simulink model "reaction_wheel"  (R2015b)
settings: Solver=VariableStepAuto  StartTime=0.0  StopTime=500  FixedStep=0.0005  RelTol=1e-3
settings Model: Creator=150010037  LastModifiedBy=150010037

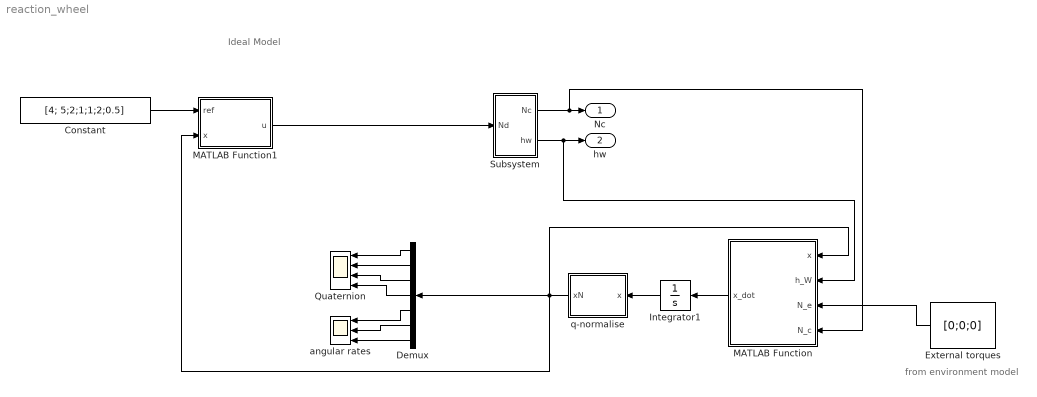
== system reaction_wheel ==
  note: Ideal Model
  note: from environment model
  Constant : Constant  Value=[4; 5;2;1;1;2;0.5]
  Demux : Demux  Outputs=7
  "External torques " : Constant  Value=[0;0;0]
  Integrator1 : Integrator  InitialCondition=[2;3;5;3;0.23;0.5;0.001]
  MATLAB Function : MATLAB Function  TreatAsAtomicUnit=on
  MATLAB Function1 : MATLAB Function  TreatAsAtomicUnit=on
  Quaternion : Scope  NumInputPorts=4
  Subsystem : Subsystem
  angular rates : Scope  NumInputPorts=3
  q-normalise : MATLAB Function  TreatAsAtomicUnit=on
  Nc : Outport
  "hw " : Outport  Port=2
  wires:
  MATLAB Function/1(x_dot) -> Integrator1/1
  Integrator1/1 -> q-normalise/1(x)
  q-normalise/1(xN) -> MATLAB Function1/2(x), MATLAB Function/1(x), Demux/1
  Subsystem/1(Nc) -> MATLAB Function/4(N_c), Nc/1
  Subsystem/2("hw ") -> MATLAB Function/2(h_W), "hw "/1
  "External torques "/1 -> MATLAB Function/3(N_e)
  MATLAB Function1/1(u) -> Subsystem/1(Nd)
  Demux/4 -> Quaternion/4
  Demux/1 -> Quaternion/1
  Demux/2 -> Quaternion/2
  Demux/3 -> Quaternion/3
  Demux/6 -> angular rates/2
  Demux/5 -> angular rates/1
  Demux/7 -> angular rates/3
  Constant/1 -> MATLAB Function1/1(ref)

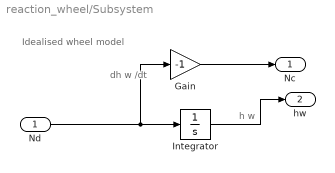
== system reaction_wheel/Subsystem ==
  note: Idealised wheel
      | model
  note: dh w /dt
  note: h w
  Nd : Inport
  Gain : Gain  Gain=-1
  Integrator : Integrator  InitialCondition=[0;0;0]
  Nc : Outport
  "hw " : Outport  Port=2
  wires:
  Nd/1 -> Gain/1, Integrator/1
  Integrator/1 -> "hw "/1
  Gain/1 -> Nc/1

== matlab function reaction_wheel/MATLAB Function1 ==
  data: ref input; x input; u output
function u = fcn(ref,x)
r=ref;
%quaternion error calculation
q_ref=[r(4) r(3) -r(2) -r(1) ;-r(3) r(4) r(1) r(2);r(2) -r(1) r(4) -r(3);r(1) r(2) r(3) r(4)];
q_s=x(1:4);
q_e=q_ref * q_s;
q1_e=[q_e(1)*q_e(4);q_e(2)*q_e(4);q_e(3)*q_e(4)];
%angular velocity error calculation
w_s=x(5:7);
w_r=r(5:7);
w_e=w_s -w_r;
kp=0.002; kpd =0.001;
u=-kp*q1_e - kpd*w_e;

== matlab function reaction_wheel/MATLAB Function ==
  data: x input; x_dot output; h_W input; N_e input; N_c input
function x_dot= fcn(x,h_W,N_e,N_c)
%W_dot calculation
w = x(5:7);
S_W=[ 0 -w(3) w(2);w(3) 0 w(1);-w(2) w(1) 0;];
I_s=[14.3 0 0;0 13.6 0; 0 0 4.6 ];
%I_s=[0 0 1.1;0 1.1 0; 0 0 1.1 ];
w_dot=-I_s\S_W*I_s*w - I_s\S_W*h_W + I_s\N_c + I_s\N_e;      %I_s\ means inv(I_s)*Ne

%q_dot calculation
q = x(1:4);
W = ...
    [ 0 w(3) -w(2) w(1);
      -w(3) 0 w(1) w(2);
      w(2) -w(1) 0 w(3);
      -w(1) -w(2) -w(3) 0];
  
q_dot = 0.5 * W * q;
x_dot=[q_dot;w_dot];

== matlab function reaction_wheel/q-normalise ==
  data: x input; xN output
function xN  = fcn(x)

q = x(1:4);
q = q/sqrt(dot(q,q));
xN = [q; x(5:7)];
